simulink model "Stateflow_Arduino__Uno"  (R2021b)
settings: Solver=VariableStepAuto  StartTime=0.0  StopTime=120  RelTol=1e-3
model workspace (MAT data in the model file):
  courseObject.course = 'stateflow'
  courseObject.chapter = 10
  courseObject.lesson = 1
  courseObject.section = 2
  courseObject.task = 1
CloseFcn:
  | learning.simulink.cleanupOnlineTraining
settings Model: Creator=Jeedella  LastModifiedBy=Jeedella
settings DataIOCC: SaveTime=off

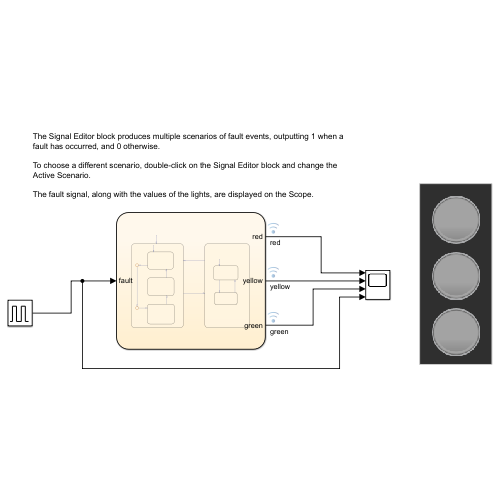
[thumbnail: Simulink's stored preview of the top-level diagram]
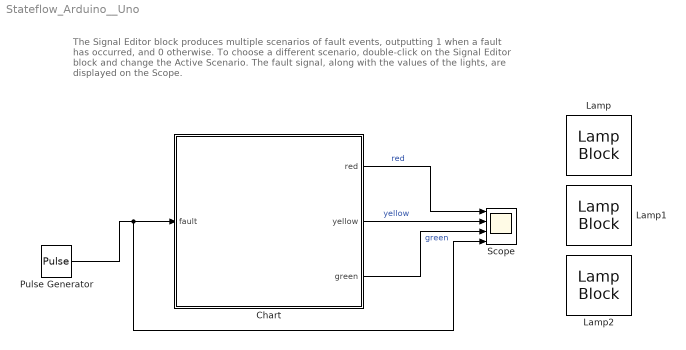
== system Stateflow_Arduino__Uno ==
  note: The Signal Editor block produces multiple scenarios of fault events, outputting 1 when a fault has occurred, and 0 otherwise.
      |
      | To choose a different scenario, double-click on the Signal Editor block and change the Active Scenario.
      |
      | The fault signal, along with the values of the lights, are displayed on the Scope.
  Chart : Stateflow chart  TreatAsAtomicUnit=on
  Lamp : LampBlock  LabelPosition=Hide
  Lamp1 : LampBlock  LabelPosition=Hide
  Lamp2 : LampBlock  LabelPosition=Hide
  Pulse Generator : DiscretePulseGenerator  PulseType=Time based  Period=60
  Scope : Scope  NumInputPorts=4
  wires:
  Chart/2(yellow) -> Scope/2  "yellow"
  Chart/3(green) -> Scope/3  "green"
  Chart/1(red) -> Scope/1  "red"
  Pulse Generator/1 -> Scope/4, Chart/1(fault)

== stateflow chart Stateflow_Arduino__Uno/Chart ==
  state Normal
    state Stop
      entry:
      red = 1;
      yellow = 0;
      green = 0;
    state PrepareToStop
      entry:
      red = 0;
      yellow = 1;
      green = 0;
    state Go
      entry:
      red = 0;
      yellow = 0;
      green = 1;
    (default) -> Stop
    Stop -> (junction 26)
    (junction 26) -> (junction 29) : after(3,sec)
    PrepareToStop -> Stop : after(3,sec)
    Go -> PrepareToStop : after(10,sec)
    (junction 29) -> Go
  state Fault
    entry:
    yellow = 0;
    green = 0;
    state BlinkOn
      during:
      red = 1;
    state BlinkOff
      during:
      red = 0;
    (default) -> BlinkOn
    BlinkOn -> BlinkOff : after(3,sec)
    BlinkOff -> BlinkOn : after(3,sec)
  (default) -> Normal
  Fault -> Normal : [fault == 0]
  Normal -> Fault : [fault == 1]
  data: red output =1; yellow output; fault input; green output =0
